simulink model "test_NCO"  (R2019b)
settings: Solver=FixedStepAuto  StartTime=0.0  StopTime=0.001  FixedStep=1/26e6  RelTol=1e-3
libraries: dspsigops x1, simulink x1
settings Model: Creator=nishantmittal  LastModifiedBy=nishantmittal

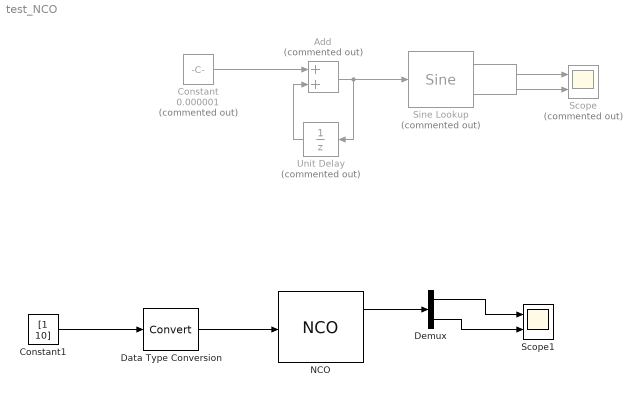
== system test_NCO ==
  Add : Sum  Commented=on
  Constant : Constant  Commented=on  Value=0.000001
  Constant1 : Constant  Value=[1 10]
  Data Type Conversion : DataTypeConversion
  Demux : Demux  Outputs=2
  NCO : dspsigops/NCO  AccIncSrc=Input port  AccInc=1  PhaseOffsetSrc=Specify via dialog  PhaseOffset=[0 0]  AccumWL=16  HasDither=off  DitherWL=15  PNgeneratorLength=19  HasPhaseQuantizer=off  TableDepth=15  HasOutputPhaseError=off  Formula=Sine and cosine  DataType=Binary point scaling  OutputWL=16  OutputFL=14  CompMethod=Table lookup (no interpolation)  SampleTime=1/1e6  SamplesPerFrame=1  OutputFrames=off
      settings: SourceProductName=DSP System Toolbox  SourceProductBaseCode=DS
  Scope : Scope  Commented=on  NumInputPorts=2
  Scope1 : Scope  NumInputPorts=2
  Sine Lookup : simulink/Lookup Tables/Sine  Commented=on  Formula=sin(2*pi*u) and cos(2*pi*u)  NumDataPoints=(2^10)+1  OutputWordLength=12  InternalRulePriority=Speed
      settings: SourceProductName=Simulink
  Unit Delay : UnitDelay  Commented=on  SampleTime=1/1e6  HasFrameUpgradeWarning=on
  wires:
  Sine Lookup/2 -> Scope/1
  Sine Lookup/1 -> Scope/2
  Add/1 -> Unit Delay/1, Sine Lookup/1
  Constant/1 -> Add/1
  Unit Delay/1 -> Add/2
  Constant1/1 -> Data Type Conversion/1
  Data Type Conversion/1 -> NCO/1
  NCO/1 -> Demux/1
  Demux/1 -> Scope1/1
  Demux/2 -> Scope1/2
